simulink model "simul3"  (R2021b)
settings: Solver=VariableStepAuto  StartTime=0.0  StopTime=10.0  RelTol=1e-3
settings Model: Creator=radek  LastModifiedBy=radek

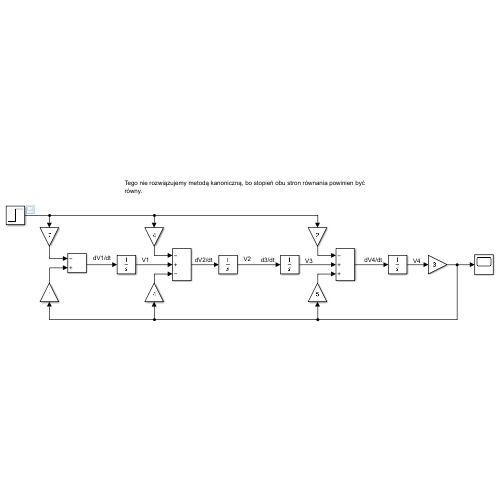
[thumbnail: Simulink's stored preview of the top-level diagram]
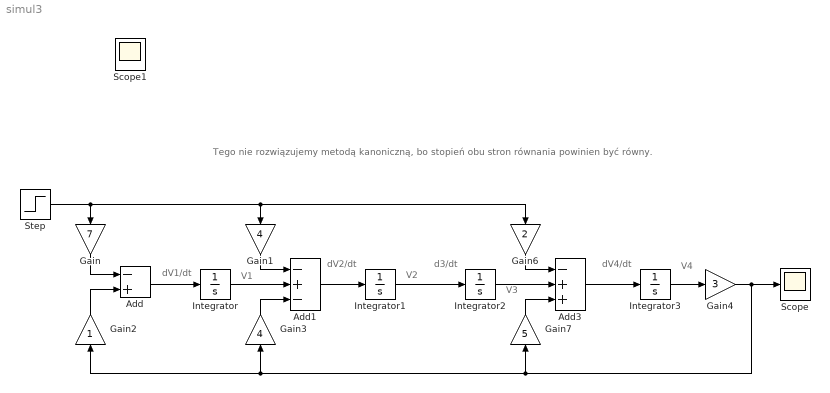
== system simul3 ==
  note: Tego nie rozwiązujemy metodą kanoniczną, bo stopień obu stron równania powinien być równy.
  note: V3
  note: V2
  note: V1
  note: dV2/dt
  note: dV1/dt
  note: d3/dt
  note: V4
  note: dV4/dt
  Add : Sum  Inputs=-+
  Add1 : Sum  Inputs=-+-
  Add3 : Sum  Inputs=-++
  Gain : Gain  Gain=7
  Gain1 : Gain  Gain=4
  Gain2 : Gain
  Gain3 : Gain  Gain=4
  Gain4 : Gain  Gain=3
  Gain6 : Gain  Gain=2
  Gain7 : Gain  Gain=5
  Integrator{,1..3} (4 alike) : Integrator
  Scope : Scope
  Step : Step  SampleTime=0
  Scope1 : Scope
  wires:
  Gain/1 -> Add/1
  Add/1 -> Integrator/1
  Gain2/1 -> Add/2
  Integrator/1 -> Add1/2
  Gain1/1 -> Add1/1
  Gain3/1 -> Add1/3
  Add1/1 -> Integrator1/1
  Gain7/1 -> Add3/3
  Gain6/1 -> Add3/1
  Integrator2/1 -> Add3/2
  Integrator3/1 -> Gain4/1
  Add3/1 -> Integrator3/1
  Step/1 -> Gain6/1, Gain1/1, Gain/1
  Gain4/1 -> Gain3/1, Gain2/1, Gain7/1, Scope/1
  Integrator1/1 -> Integrator2/1
